simulink model "Solo_M1"  (R2024b)
settings: Solver=VariableStepAuto  StartTime=0.0  StopTime=86400*2  RelTol=1e-3
values from neighbouring files (symbols this model uses):
  xk0 = zeros(36, 1)    [getinput_test.m]
settings Model: Creator=Laura  LastModifiedBy=Laura

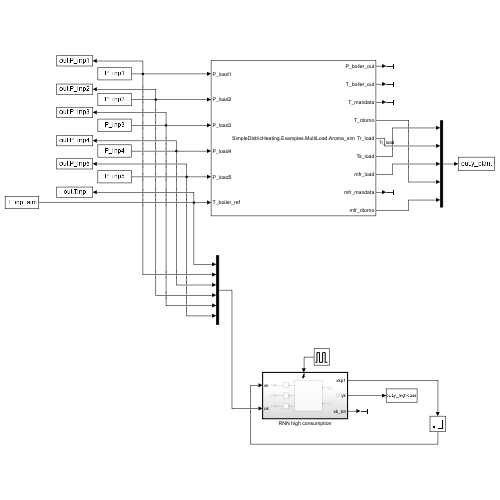
[thumbnail: Simulink's stored preview of the top-level diagram]
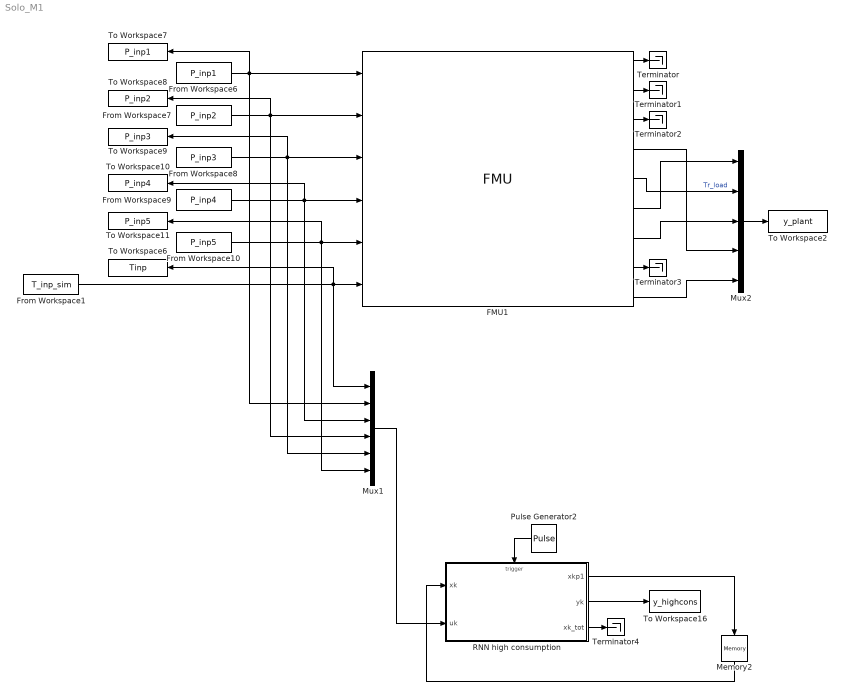
== system Solo_M1 ==
  FMU1 : FMU  FMUName=SimpleDistricHeating.Examples.MultiLoad.Aroma_sim.fmu  FMUMode=ModelExchange  FMUInitializeEnumObject=off  boiler=struct('P_max',100000000.0,'P_min',1000.0,'T_vol',353.15,'V',0.16,'boilePowerUnit',struct('b',0.001),'boilerInsideVolume',struct('T_amb',288.15,'UA',0.0,'allowFlowReversal',boolean(false)),'boilerPIControl',struct('D',struct('y_start',0.0),'FFzero',struct('k',0.0),'Nd',10.0,'Ni',0.9,'P',struct('k',1.0),'Td',0.1,'Ti',8.0,'addD',struct('k2',-1.0),'addFF',struct('k1',1.0),'addI',struct('k1',1.0,'k2',-1.0,'k3',1.0),'addP',struct('k2',-1.0),'addPID',struct('k1',1.0,'k2',1.0,'k3',1.0),'addSat',struct('k1',1.0,'k2',-1.0),'k',50000.0,'kFF',1.0,'limiter',struct('uMax',100000000.0,'uMin',1000.0),'wd',0.0,'wp',1.0,'xd_start',0.0,'xi_start',0.0),'integralTime',16.0)  load1=struct('Kv',36.0,'dp_nom',400000.0,'load',struct('b',0.001),'loadValveControl',struct('Dzero',struct('k',0.0),'FFzero',struct('k',0.0),'Izero',struct('k',0.0),'Nd',10.0,'Ni',0.9,'P',struct('k',1.0),'Td',0.1,'Ti',0.5,'addFF',struct('k1',1.0),'addP',struct('k2',-1.0),'addPID',struct('k1',1.0,'k2',1.0,'k3',1.0),'k',0.05,'kFF',1.0,'limiter',struct('uMax',1.0,'uMin',0.0),'wd',0.0,'wp',1.0,'xd_start',0.0,'xi_start',0.0),'m_nom',25.0,'theta_min',0.001,'theta_nom',1.0)  load2=struct('Kv',36.0,'dp_nom',400000.0,'load',struct('b',0.001),'loadValveControl',struct('Dzero',struct('k',0.0),'FFzero',struct('k',0.0),'Izero',struct('k',0.0),'Nd',10.0,'Ni',0.9,'P',struct('k',1.0),'Td',0.1,'Ti',0.5,'addFF',struct('k1',1.0),'addP',struct('k2',-1.0),'addPID',struct('k1',1.0,'k2',1.0,'k3',1.0),'k',0.05,'kFF',1.0,'limiter',struct('uMax',1.0,'uMin',0.0),'wd',0.0,'wp',1.0,'xd_start',0.0,'xi_start',0.0),'m_nom',25.0,'theta_min',0.001,'theta_nom',1.0)  load3=struct('Kv',36.0,'dp_nom',400000.0,'load',struct('b',0.001),'loadValveControl',struct('Dzero',struct('k',0.0),'FFzero',struct('k',0.0),'Izero',struct('k',0.0),'Nd',10.0,'Ni',0.9,'P',struct('k',1.0),'Td',0.1,'Ti',0.5,'addFF',struct('k1',1.0),'addP',struct('k2',-1.0),'addPID',struct('k1',1.0,'k2',1.0,'k3',1.0),'k',0.05,'kFF',1.0,'limiter',struct('uMax',1.0,'uMin',0.0),'wd',0.0,'wp',1.0,'xd_start',0.0,'xi_start',0.0),'m_nom',25.0,'theta_min',0.001,'theta_nom',1.0)  load4=struct('Kv',36.0,'dp_nom',400000.0,'load',struct('b',0.001),'loadValveControl',struct('Dzero',struct('k',0.0),'FFzero',struct('k',0.0),'Izero',struct('k',0.0),'Nd',10.0,'Ni',0.9,'P',struct('k',1.0),'Td',0.1,'Ti',0.5,'addFF',struct('k1',1.0),'addP',struct('k2',-1.0),'addPID',struct('k1',1.0,'k2',1.0,'k3',1.0),'k',0.05,'kFF',1.0,'limiter',struct('uMax',1.0,'uMin',0.0),'wd',0.0,'wp',1.0,'xd_start',0.0,'xi_start',0.0),'m_nom',25.0,'theta_min',0.001,'theta_nom',1.0)  load5=struct('Kv',36.0,'dp_nom',400000.0,'load',struct('b',0.001),'loadValveControl',struct('Dzero',struct('k',0.0),'FFzero',struct('k',0.0),'Izero',struct('k',0.0),'Nd',10.0,'Ni',0.9,'P',struct('k',1.0),'Td',0.1,'Ti',0.5,'addFF',struct('k1',1.0),'addP',struct('k2',-1.0),'addPID',struct('k1',1.0,'k2',1.0,'k3',1.0),'k',0.05,'kFF',1.0,'limiter',struct('uMax',1.0,'uMin',0.0),'wd',0.0,'wp',1.0,'xd_start',0.0,'xi_start',0.0),'m_nom',25.0,'theta_min',0.001,'theta_nom',1.0)  load_ref=struct('k',65.0)  pressureAccumulator=struct('T0',338.15,'p_2',499999.9999999999)  pumpDifferentialPressure=struct('dp',499999.9999999999)  r10=struct('D',0.107,'L',500.0,'T_ext',298.15,'T_start',337.15,'cf',0.004,'conductivity_pipe_ins',0.02,'dIns',0.2,'dWall',0.003,'lambda',45.0,'rhomcm',3120000.0,'u_nom',1.5)  r21=struct('D',0.107,'L',282.8,'T_ext',298.15,'T_start',337.15,'cf',0.004,'conductivity_pipe_ins',0.02,'dIns',0.2,'dWall',0.003,'lambda',45.0,'rhomcm',3120000.0,'u_nom',1.5)  r32=struct('D',0.083,'L',500.0,'T_ext',298.15,'T_start',337.15,'cf',0.004,'conductivity_pipe_ins',0.02,'dIns',0.2,'dWall',0.003,'lambda',45.0,'rhomcm',3120000.0,'u_nom',1.5)  r43=struct('D',0.083,'L',282.8,'T_ext',298.15,'T_start',337.15,'cf',0.004,'conductivity_pipe_ins',0.02,'dIns',0.2,'dWall',0.003,'lambda',45.0,'rhomcm',3120000.0,'u_nom',1.5)  r54=struct('D',0.07000000000000001,'L',400.0,'T_ext',298.15,'T_start',337.15,'cf',0.004,'conductivity_pipe_ins',0.02,'dIns',0.2,'dWall',0.003,'lambda',45.0,'rhomcm',3120000.0,'u_nom',1.5)  r61=struct('D',0.107,'L',282.8,'T_ext',298.15,'T_start',337.15,'cf',0.004,'conductivity_pipe_ins',0.02,'dIns',0.2,'dWall',0.003,'lambda',45.0,'rhomcm',3120000.0,'u_nom',1.5)  r74=struct('D',0.083,'L',282.8,'T_ext',298.15,'T_start',337.15,'cf',0.004,'conductivity_pipe_ins',0.02,'dIns',0.2,'dWall',0.003,'lambda',45.0,'rhomcm',3120000.0,'u_nom',1.5)  r76=struct('D',0.083,'L',500.0,'T_ext',298.15,'T_start',337.15,'cf',0.004,'conductivity_pipe_ins',0.02,'dIns',0.2,'dWall',0.003,'lambda',45.0,'rhomcm',3120000.0,'u_nom',1.5)  r87=struct('D',0.07000000000000001,'L',600.0,'T_ext',298.15,'T_start',337.15,'cf',0.004,'conductivity_pipe_ins',0.02,'dIns',0.2,'dWall',0.003,'lambda',45.0,'rhomcm',3120000.0,'u_nom',1.5)  s01=struct('D',0.107,'L',500.0,'T_ext',298.15,'T_start',353.15,'cf',0.004,'conductivity_pipe_ins',0.02,'dIns',0.2,'dWall',0.003,'lambda',45.0,'rhomcm',3120000.0,'u_nom',1.5)  s12=struct('D',0.107,'L',282.8,'T_ext',298.15,'T_start',353.15,'cf',0.004,'conductivity_pipe_ins',0.02,'dIns',0.2,'dWall',0.003,'lambda',45.0,'rhomcm',3120000.0,'u_nom',1.5)  s16=struct('D',0.107,'L',282.8,'T_ext',298.15,'T_start',353.15,'cf',0.004,'conductivity_pipe_ins',0.02,'dIns',0.2,'dWall',0.003,'lambda',45.0,'rhomcm',3120000.0,'u_nom',1.5)  s23=struct('D',0.083,'L',500.0,'T_ext',298.15,'T_start',353.15,'cf',0.004,'conductivity_pipe_ins',0.02,'dIns',0.2,'dWall',0.003,'lambda',45.0,'rhomcm',3120000.0,'u_nom',1.5)  s34=struct('D',0.083,'L',282.8,'T_ext',298.15,'T_start',353.15,'cf',0.004,'conductivity_pipe_ins',0.02,'dIns',0.2,'dWall',0.003,'lambda',45.0,'rhomcm',3120000.0,'u_nom',1.5)  s45=struct('D',0.07000000000000001,'L',400.0,'T_ext',298.15,'T_start',353.15,'cf',0.004,'conductivity_pipe_ins',0.02,'dIns',0.2,'dWall',0.003,'lambda',45.0,'rhomcm',3120000.0,'u_nom',1.5)  s47=struct('D',0.083,'L',282.8,'T_ext',298.15,'T_start',353.15,'cf',0.004,'conductivity_pipe_ins',0.02,'dIns',0.2,'dWall',0.003,'lambda',45.0,'rhomcm',3120000.0,'u_nom',1.5)  s67=struct('D',0.083,'L',500.0,'T_ext',298.15,'T_start',353.15,'cf',0.004,'conductivity_pipe_ins',0.02,'dIns',0.2,'dWall',0.003,'lambda',45.0,'rhomcm',3120000.0,'u_nom',1.5)  s78=struct('D',0.07000000000000001,'L',600.0,'T_ext',298.15,'T_start',353.15,'cf',0.004,'conductivity_pipe_ins',0.02,'dIns',0.2,'dWall',0.003,'lambda',45.0,'rhomcm',3120000.0,'u_nom',1.5)  mask(SimpleDistricHeating.Examples.MultiLoad.Aroma_sim [Model Exchange, v2.0]){}
      settings: MultithreadedSim=off
      mask Display:
      | disp('SimpleDistricHeating.Examples.MultiLoad.Aroma_sim');
      | port_label('output',1,'P_boiler_out');
      | port_label('output',2,'T_boiler_out');
      | port_label('output',3,'T_mandata');
      | port_label('output',4,'T_ritorno');
      | port_label('output',5,'Tr_load');
      | port_label('output',6,'Ts_load');
      | port_label('output',7,'mfr_load');
      | port_label('output',8,'mfr_mandata');
      | port_label('output',9,'mfr_ritorno');
      | port_label('input',1,'P_load1');
      | port_label('input',2,'P_load2');
      | port_label('input',3,'P_load3');
      | port_label('input',4,'P_load4');
      | port_label('input',5,'P_load5');
      | port_label('input',6,'T_boiler_ref');
  From Workspace1 : FromWorkspace  VariableName=T_inp_sim  SampleTime=-1
  From Workspace10 : FromWorkspace  VariableName=P_inp5  SampleTime=-1
  From Workspace6 : FromWorkspace  VariableName=P_inp1  SampleTime=-1
  From Workspace7 : FromWorkspace  VariableName=P_inp2  SampleTime=-1
  From Workspace8 : FromWorkspace  VariableName=P_inp3  SampleTime=-1
  From Workspace9 : FromWorkspace  VariableName=P_inp4  SampleTime=-1
  Memory2 : Memory  InitialCondition=xk0
  Mux1 : Mux  Inputs=6
  Mux2 : Mux  Inputs=5
  Pulse Generator2 : DiscretePulseGenerator  PulseType=Time based  Period=300  PulseWidth=5
  RNN high consumption : Subsystem  TreatAsAtomicUnit=on
  Terminator{,1..4} (5 alike) : Terminator
  To Workspace10 : ToWorkspace  VariableName=P_inp4  SampleTime=300
  To Workspace11 : ToWorkspace  VariableName=P_inp5  SampleTime=300
  To Workspace16 : ToWorkspace  VariableName=y_highcons  SampleTime=300
  To Workspace2 : ToWorkspace  VariableName=y_plant  SampleTime=300
  To Workspace6 : ToWorkspace  VariableName=Tinp  SampleTime=300
  To Workspace7 : ToWorkspace  VariableName=P_inp1  SampleTime=300
  To Workspace8 : ToWorkspace  VariableName=P_inp2  SampleTime=300
  To Workspace9 : ToWorkspace  VariableName=P_inp3  SampleTime=300
  wires:
  Mux2/1 -> To Workspace2/1
  From Workspace9/1 -> FMU1/4, Mux1/3, To Workspace10/1
  From Workspace1/1 -> FMU1/6, Mux1/1, To Workspace6/1
  RNN high consumption/2(yk) -> To Workspace16/1
  Memory2/1 -> RNN high consumption/1(xk)
  From Workspace6/1 -> FMU1/1, Mux1/2, To Workspace7/1
  From Workspace8/1 -> FMU1/3, Mux1/5, To Workspace9/1
  From Workspace10/1 -> FMU1/5, Mux1/6, To Workspace11/1
  From Workspace7/1 -> FMU1/2, Mux1/4, To Workspace8/1
  RNN high consumption/1(xkp1) -> Memory2/1
  RNN high consumption/3(xk_tot) -> Terminator4/1
  Mux1/1 -> RNN high consumption/2(uk)
  Pulse Generator2/1 -> RNN high consumption/Trigger
  FMU1/1 -> Terminator/1
  FMU1/2 -> Terminator1/1
  FMU1/3 -> Terminator2/1
  FMU1/4 -> Mux2/4
  FMU1/9 -> Mux2/5
  FMU1/8 -> Terminator3/1
  FMU1/6 -> Mux2/1
  FMU1/5 -> Mux2/2  "Tr_load"
  FMU1/7 -> Mux2/3

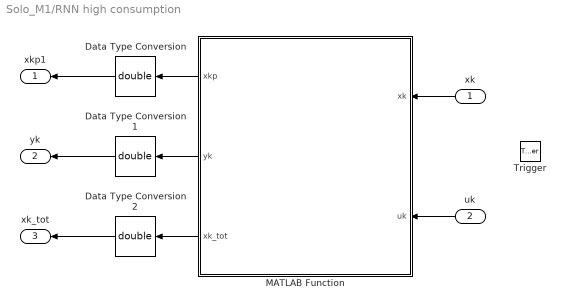
== system Solo_M1/RNN high consumption ==
  xk : Inport
  uk : Inport  Port=2
  Trigger : TriggerPort  VariantControl=(inherit)
  Data Type Conversion : DataTypeConversion  OutDataTypeStr=double  RndMeth=Nearest  SaturateOnIntegerOverflow=off
  Data Type Conversion1 : DataTypeConversion  OutDataTypeStr=double  RndMeth=Nearest  SaturateOnIntegerOverflow=off
  Data Type Conversion2 : DataTypeConversion  OutDataTypeStr=double  RndMeth=Nearest  SaturateOnIntegerOverflow=off
  MATLAB Function : MATLAB Function  TreatAsAtomicUnit=on
  xkp1 : Outport
  yk : Outport  Port=2
  xk_tot : Outport  Port=3
  wires:
  xk/1 -> MATLAB Function/1(xk)
  uk/1 -> MATLAB Function/2(uk)
  MATLAB Function/2(yk) -> Data Type Conversion1/1
  MATLAB Function/1(xkp) -> Data Type Conversion/1
  Data Type Conversion/1 -> xkp1/1
  Data Type Conversion1/1 -> yk/1
  Data Type Conversion2/1 -> xk_tot/1
  MATLAB Function/3(xk_tot) -> Data Type Conversion2/1

== matlab function Solo_M1/RNN high consumption/MATLAB Function ==
  data: xkp output; xk input; uk input; yk output; xk_tot output
function [xkp, yk, xk_tot] = RNN(xk, uk)

    n_states = [2,2,2,4,3,5];
    layers_file = load("layers_file_highconsumption.mat");
    input_scaler_file = load("input_scaler_file_highconsumption.mat");
    output_scaler_file = load("output_scaler_file_highconsumption.mat");
    
    layers_file = layers_file.layers_file;
    input_scaler_file = input_scaler_file.input_scaler_file;
    output_scaler_file = output_scaler_file.output_scaler_file;

    % Scale input
    uk = (uk  - (input_scaler_file.input_scaler.bias).') ./ (input_scaler_file.input_scaler.scale).';

    % Sum of powers
    sum1 = uk(3,:)+uk(4,:)+uk(5,:)+uk(6,:);
    sum2 = uk(2,:)+uk(4,:)+uk(5,:)+uk(6,:);
    sum3 = uk(2,:)+uk(3,:)+uk(5,:)+uk(6,:);
    sum4 = uk(2,:)+uk(3,:)+uk(4,:)+uk(6,:);
    sum5 = uk(2,:)+uk(3,:)+uk(4,:)+uk(5,:);
    
    % GRU 1
    uk1 = [uk(1,:); uk(2,:); sum1];
    xk1 = xk(1:n_states(1),:);    
    zk1 = sigmoidfunction((layers_file.layers{1,1}.weights.Wzf(:,1:n_states(1))).' * uk1 + (layers_file.layers{1,1}.weights.Uzf(:,1:n_states(1))).' * xk1 + (layers_file.layers{1,1}.weights.bzf(:,1:n_states(1))).');
    fk1 = sigmoidfunction((layers_file.layers{1,1}.weights.Wzf(:,n_states(1)+1:end)).' * uk1 + (layers_file.layers{1,1}.weights.Uzf(:,n_states(1)+1:end)).' * xk1 + (layers_file.layers{1,1}.weights.bzf(:,n_states(1)+1:end)).');
    phi1 = tanh((layers_file.layers{1,1}.weights.Wr).' * uk1 + (layers_file.layers{1,1}.weights.Ur).' * (fk1.* xk1) + (layers_file.layers{1,1}.weights.br).');
    xkp1 = zk1 .* xk1 + (1-zk1) .* phi1;
    yk1 = layers_file.layers{1,2}.weights.weight * xk1 + (layers_file.layers{1,2}.weights.bias).';
    
    % GRU 2
    uk2 = [uk(1,:); uk(3,:); sum2];
    xk2 = xk(n_states(1)+1:n_states(1)+n_states(2),:);
    zk2 = sigmoidfunction((layers_file.layers{1,3}.weights.Wzf(:,1:n_states(2))).' * uk2 + (layers_file.layers{1,3}.weights.Uzf(:,1:n_states(2))).' * xk2 + (layers_file.layers{1,3}.weights.bzf(:,1:n_states(2))).');
    fk2 = sigmoidfunction((layers_file.layers{1,3}.weights.Wzf(:,n_states(2)+1:end)).' * uk2 + (layers_file.layers{1,3}.weights.Uzf(:,n_states(2)+1:end)).' * xk2 + (layers_file.layers{1,3}.weights.bzf(:,n_states(2)+1:end)).');
    phi2 = tanh((layers_file.layers{1,3}.weights.Wr).' * uk2 + (layers_file.layers{1,3}.weights.Ur).' * (fk2.* xk2) + (layers_file.layers{1,3}.weights.br).');
    xkp2 = zk2 .* xk2 + (1-zk2) .* phi2;
    yk2 = layers_file.layers{1,4}.weights.weight * xk2 + (layers_file.layers{1,4}.weights.bias).';
    
    % GRU 3
    uk3 = [uk(4,:); yk1(1,:); sum3];
    xk3 = xk(n_states(1)+n_states(2)+1:n_states(1)+n_states(2)+n_states(3),:);
    zk3 = sigmoidfunction((layers_file.layers{1,5}.weights.Wzf(:,1:n_states(3))).' * uk3 + (layers_file.layers{1,5}.weights.Uzf(:,1:n_states(3))).' * xk3 + (layers_file.layers{1,5}.weights.bzf(:,1:n_states(3))).');
    fk3 = sigmoidfunction((layers_file.layers{1,5}.weights.Wzf(:,n_states(3)+1:end)).' * uk3 + (layers_file.layers{1,5}.weights.Uzf(:,n_states(3)+1:end)).' * xk3 + (layers_file.layers{1,5}.weights.bzf(:,n_states(3)+1:end)).');
    phi3 = tanh((layers_file.layers{1,5}.weights.Wr).' * uk3 + (layers_file.layers{1,5}.weights.Ur).' * (fk3.* xk3) + (layers_file.layers{1,5}.weights.br).');
    xkp3 = zk3 .* xk3 + (1-zk3) .* phi3;
    yk3 = layers_file.layers{1,6}.weights.weight * xk3 + (layers_file.layers{1,6}.weights.bias).';
    
    % GRU 4
    uk4 = [uk(5,:); yk2(1,:); yk3(1,:); sum4];
    xk4 = xk(n_states(1)+n_states(2)+n_states(3)+1:n_states(1)+n_states(2)+n_states(3)+n_states(4),:);
    zk4 = sigmoidfunction((layers_file.layers{1,7}.weights.Wzf(:,1:n_states(4))).' * uk4 + (layers_file.layers{1,7}.weights.Uzf(:,1:n_states(4))).' * xk4 + (layers_file.layers{1,7}.weights.bzf(:,1:n_states(4))).');
    fk4 = sigmoidfunction((layers_file.layers{1,7}.weights.Wzf(:,n_states(4)+1:end)).' * uk4 + (layers_file.layers{1,7}.weights.Uzf(:,n_states(4)+1:end)).' * xk4 + (layers_file.layers{1,7}.weights.bzf(:,n_states(4)+1:end)).');
    phi4 = tanh((layers_file.layers{1,7}.weights.Wr).' * uk4 + (layers_file.layers{1,7}.weights.Ur).' * (fk4.* xk4) + (layers_file.layers{1,7}.weights.br).');
    xkp4 = zk4 .* xk4 + (1-zk4) .* phi4;
    yk4 = layers_file.layers{1,8}.weights.weight * xk4 + (layers_file.layers{1,8}.weights.bias).';

    % GRU 5
    uk5 = [uk(6,:); yk2(1,:); yk3(1,:); sum5];
    xk5 = xk(n_states(1)+n_states(2)+n_states(3)+n_states(4)+1:n_states(1)+n_states(2)+n_states(3)+n_states(4)+n_states(5),:);
    zk5 = sigmoidfunction((layers_file.layers{1,9}.weights.Wzf(:,1:n_states(5))).' * uk5 + (layers_file.layers{1,9}.weights.Uzf(:,1:n_states(5))).' * xk5 + (layers_file.layers{1,9}.weights.bzf(:,1:n_states(5))).');
    fk5 = sigmoidfunction((layers_file.layers{1,9}.weights.Wzf(:,n_states(5)+1:end)).' * uk5 + (layers_file.layers{1,9}.weights.Uzf(:,n_states(5)+1:end)).' * xk5 + (layers_file.layers{1,9}.weights.bzf(:,n_states(5)+1:end)).');
    phi5 = tanh((layers_file.layers{1,9}.weights.Wr).' * uk5 + (layers_file.layers{1,9}.weights.Ur).' * (fk5.* xk5) + (layers_file.layers{1,9}.weights.br).');
    xkp5 = zk5 .* xk5 + (1-zk5) .* phi5;
    yk5 = layers_file.layers{1,10}.weights.weight * xk5 + (layers_file.layers{1,10}.weights.bias).';

    % GRU 6
    uk6 = [yk1(2,:); yk1(3,:); yk2(2,:); yk2(3,:); yk3(2,:); yk3(3,:); yk4(2,:); yk4(3,:); yk5(2,:); yk5(3,:)];
    xk6 = xk(n_states(1)+n_states(2)+n_states(3)+n_states(4)+n_states(5)+1:n_states(1)+n_states(2)+n_states(3)+n_states(4)+n_states(5)+n_states(6),:);
    zk6 = sigmoidfunction((layers_file.layers{1,11}.weights.Wzf(:,1:n_states(6))).' * uk6 + (layers_file.layers{1,11}.weights.Uzf(:,1:n_states(6))).' * xk6 + (layers_file.layers{1,11}.weights.bzf(:,1:n_states(6))).');
    fk6 = sigmoidfunction((layers_file.layers{1,11}.weights.Wzf(:,n_states(6)+1:end)).' * uk6 + (layers_file.layers{1,11}.weights.Uzf(:,n_states(6)+1:end)).' * xk6 + (layers_file.layers{1,11}.weights.bzf(:,n_states(6)+1:end)).');
    phi6 = tanh((layers_file.layers{1,11}.weights.Wr).' * uk6 + (layers_file.layers{1,11}.weights.Ur).' * (fk6.* xk6) + (layers_file.layers{1,11}.weights.br).');
    xkp6 = zk6 .* xk6 + (1-zk6) .* phi6;
    yk6 = layers_file.layers{1,12}.weights.weight * xk6 + (layers_file.layers{1,12}.weights.bias).';
    
    % Overall
    xk_tot = [xk1; xk2; xk3; xk4; xk5; xk6];
    xkp = [xkp1; xkp2; xkp3; xkp4; xkp5; xkp6];
    yk = [yk1; yk2; yk3; yk4; yk5; yk6];
    yk = yk .* (output_scaler_file.output_scaler.scale).' + (output_scaler_file.output_scaler.bias).';
end
